simulink model "week3_problem3"  (R2020b)
settings: Solver=VariableStepAuto  StartTime=0.0  StopTime=10.0  RelTol=1e-3
model workspace (MAT data in the model file):
  Iyy = 2100
  Lf = 0.9
  Lr = 1.2
  Mb = 1200
  cf = 2500
  cr = 2000
  kf = 28000
  kr = 21000
  x0 = [-4.33578832873e-18; -0.12012244898; 6.46234853557e-27; -1.03397576569e-25]
settings Model: Creator=gokul  LastModifiedBy=gokul

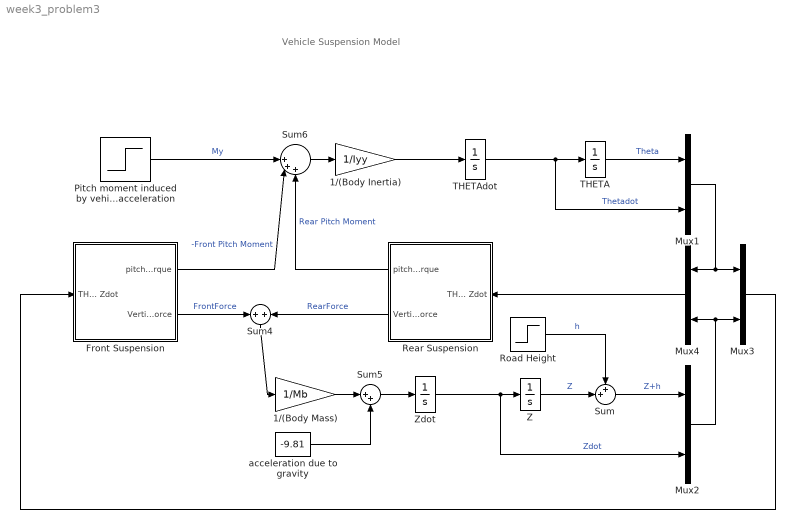
== system week3_problem3 ==
  note: Vehicle Suspension Model
  1/(Body Inertia) : Gain  Gain=1/Iyy  SaturateOnIntegerOverflow=on  OutDataTypeStr=Inherit: Same as input  ParamDataTypeStr=Inherit: Same as input
  1/(Body Mass) : Gain  Gain=1/Mb  SaturateOnIntegerOverflow=on  OutDataTypeStr=Inherit: Same as input  ParamDataTypeStr=Inherit: Same as input
  Front Suspension : Subsystem  mask(half-car suspension){K=kf, C=cf, L=-Lf}
      mask prompts: K "Stiffness = spring rate:"; C "Damping rate:"; L "Moment arm:"
      mask help:
      | Half-Car Suspension
      | The spring and damping rates for an individual wheel are entered below.  Their combined effect as applied to two wheels at the specified distance from the center of mass is computed.  The distance should be specified as positive if the subsystem is oriented such that increasing z corresponds to increasing theta, negative otherwise.
      mask Help: See "Using Simulink and Stateflow in Automotive Applications" for a mathematical derivation of the subsystem operation.  Contact your MathWorks distributor to obtain a copy.
      mask Display: plot(-1, 0, 13, 12, [1 12], [11 11], [1 5], [2 2], [1 2], [4.5 5], [2 0], [5 6], [0 2], [6 7], [2 0], [7 8], [0 1], [8 8.5], [1 1], [8.5 11], [1 1], [2 4.5], [5 5], [2 5], [4 6], [5 5], [4 4], [5 8], [6 6], [5 8], [4 6], [6.5 6.5], [5 5], [6.5 11], [0 1], [1 2], [2 3], [1 2], [4 5], [1 2])
  Mux{1..4} (4 alike) : Mux  Inputs=2
      settings: DisplayOption=signals
  Pitch moment induced by vehicle acceleration : Step  Time=3  After=100  SampleTime=0
  Rear Suspension : Subsystem  mask(half-car suspension){K=kr, C=cr, L=Lr}
      mask prompts: K "Stiffness = spring rate:"; C "Damping rate:"; L "Moment arm:"
      mask help:
      | Half-Car Suspension
      | The spring and damping rates for an individual wheel are entered below.  Their combined effect as applied to two wheels at the specified distance from the center of mass is computed.  The distance should be specified as positive if the subsystem is oriented such that increasing z corresponds to increasing theta, negative otherwise.
      mask Help: See "Using Simulink and Stateflow in Automotive Applications" for a mathematical derivation of the subsystem operation.  Contact your MathWorks distributor to obtain a copy.
      mask Display: plot(-1, 0, 13, 12, [1 12], [11 11], [1 5], [2 2], [1 2], [4.5 5], [2 0], [5 6], [0 2], [6 7], [2 0], [7 8], [0 1], [8 8.5], [1 1], [8.5 11], [1 1], [2 4.5], [5 5], [2 5], [4 6], [5 5], [4 4], [5 8], [6 6], [5 8], [4 6], [6.5 6.5], [5 5], [6.5 11], [0 1], [1 2], [2 3], [1 2], [4 5], [1 2])
  Road Height : Step  Time=7  After=0.01  SampleTime=0
  Sum : Sum  Inputs=++|
  Sum4 : Sum  InputSameDT=on  SaturateOnIntegerOverflow=on  OutDataTypeStr=Inherit: Same as first input
  Sum5 : Sum  Inputs=|++  InputSameDT=on  SaturateOnIntegerOverflow=on  OutDataTypeStr=Inherit: Same as first input
  Sum6 : Sum  Inputs=||+++  InputSameDT=on  SaturateOnIntegerOverflow=on  OutDataTypeStr=Inherit: Same as first input
  THETA : Integrator  InitialCondition=-8.7e-20
  THETAdot : Integrator  InitialCondition=8.04e-28
  Z : Integrator  InitialCondition=-0.12
  Zdot : Integrator
  acceleration due to gravity : Constant  Value=-9.81
  wires:
  Pitch moment induced by vehicle acceleration/1 -> Sum6/1  "My"
  Mux1/1 -> Mux3/1, Mux4/1
  Mux3/1 -> Front Suspension/1(THETA THETAdot Z Zdot)
  Road Height/1 -> Sum/1  "h"
  THETAdot/1 -> THETA/1, Mux1/2  "Thetadot"
  Z/1 -> Sum/2  "Z"
  Sum/1 -> Mux2/1  "Z+h"
  1/(Body Inertia)/1 -> THETAdot/1
  Mux2/1 -> Mux4/2, Mux3/2
  Sum5/1 -> Zdot/1
  Front Suspension/1(pitch Torque) -> Sum6/2  "-Front Pitch Moment"
  Mux4/1 -> Rear Suspension/1(THETA THETAdot Z Zdot)
  acceleration due to gravity/1 -> Sum5/2
  Rear Suspension/1(pitch Torque) -> Sum6/3  "Rear Pitch Moment"
  THETA/1 -> Mux1/1  "Theta"
  Front Suspension/2(Vertical Force) -> Sum4/1  "FrontForce"
  Sum6/1 -> 1/(Body Inertia)/1
  Zdot/1 -> Z/1, Mux2/2  "Zdot"
  1/(Body Mass)/1 -> Sum5/1
  Sum4/1 -> 1/(Body Mass)/1
  Rear Suspension/2(Vertical Force) -> Sum4/2  "RearForce"

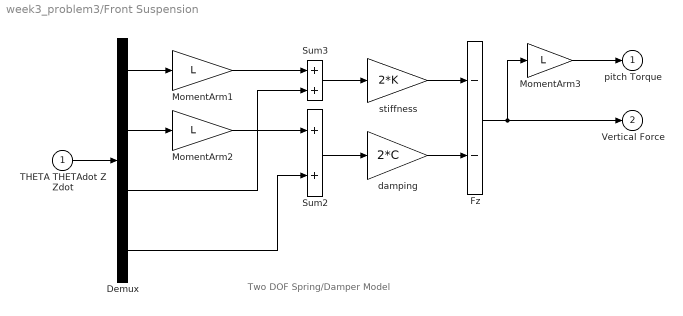
== system week3_problem3/Front Suspension ==
  note: Two DOF Spring/Damper Model
  THETA THETAdot Z Zdot : Inport
  Demux : Demux
      settings: DisplayOption=none
  Fz : Sum  Inputs=--  InputSameDT=on  SaturateOnIntegerOverflow=on  OutDataTypeStr=Inherit: Same as first input
  MomentArm1 : Gain  Gain=L  SaturateOnIntegerOverflow=on  OutDataTypeStr=Inherit: Same as input  ParamDataTypeStr=Inherit: Same as input
  MomentArm2 : Gain  Gain=L  SaturateOnIntegerOverflow=on  OutDataTypeStr=Inherit: Same as input  ParamDataTypeStr=Inherit: Same as input
  MomentArm3 : Gain  Gain=L  SaturateOnIntegerOverflow=on  OutDataTypeStr=Inherit: Same as input  ParamDataTypeStr=Inherit: Same as input
  Sum2 : Sum  InputSameDT=on  SaturateOnIntegerOverflow=on  OutDataTypeStr=Inherit: Same as first input
  Sum3 : Sum  InputSameDT=on  SaturateOnIntegerOverflow=on  OutDataTypeStr=Inherit: Same as first input
  damping : Gain  Gain=2*C  SaturateOnIntegerOverflow=on  OutDataTypeStr=Inherit: Same as input  ParamDataTypeStr=Inherit: Same as input
  stiffness : Gain  Gain=2*K  SaturateOnIntegerOverflow=on  OutDataTypeStr=Inherit: Same as input  ParamDataTypeStr=Inherit: Same as input
  pitch Torque : Outport  VectorParamsAs1DForOutWhenUnconnected=off
  Vertical Force : Outport  Port=2  VectorParamsAs1DForOutWhenUnconnected=off
  wires:
  Sum2/1 -> damping/1
  Sum3/1 -> stiffness/1
  THETA THETAdot Z Zdot/1 -> Demux/1
  damping/1 -> Fz/2
  stiffness/1 -> Fz/1
  Fz/1 -> Vertical Force/1, MomentArm3/1
  MomentArm3/1 -> pitch Torque/1
  Demux/1 -> MomentArm1/1
  Demux/2 -> MomentArm2/1
  Demux/3 -> Sum3/2
  MomentArm1/1 -> Sum3/1
  MomentArm2/1 -> Sum2/1
  Demux/4 -> Sum2/2

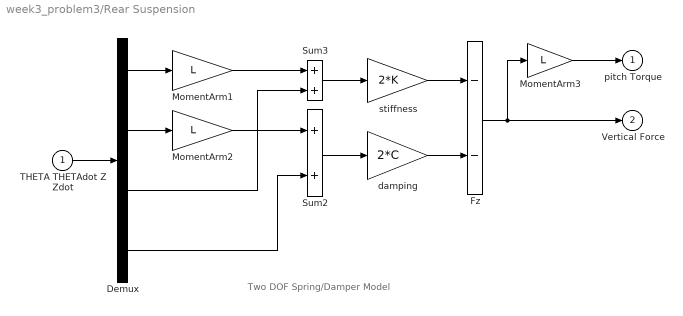
== system week3_problem3/Rear Suspension ==
  note: Two DOF Spring/Damper Model
  THETA THETAdot Z Zdot : Inport
  Demux : Demux
      settings: DisplayOption=none
  Fz : Sum  Inputs=--  InputSameDT=on  SaturateOnIntegerOverflow=on  OutDataTypeStr=Inherit: Same as first input
  MomentArm1 : Gain  Gain=L  SaturateOnIntegerOverflow=on  OutDataTypeStr=Inherit: Same as input  ParamDataTypeStr=Inherit: Same as input
  MomentArm2 : Gain  Gain=L  SaturateOnIntegerOverflow=on  OutDataTypeStr=Inherit: Same as input  ParamDataTypeStr=Inherit: Same as input
  MomentArm3 : Gain  Gain=L  SaturateOnIntegerOverflow=on  OutDataTypeStr=Inherit: Same as input  ParamDataTypeStr=Inherit: Same as input
  Sum2 : Sum  InputSameDT=on  SaturateOnIntegerOverflow=on  OutDataTypeStr=Inherit: Same as first input
  Sum3 : Sum  InputSameDT=on  SaturateOnIntegerOverflow=on  OutDataTypeStr=Inherit: Same as first input
  damping : Gain  Gain=2*C  SaturateOnIntegerOverflow=on  OutDataTypeStr=Inherit: Same as input  ParamDataTypeStr=Inherit: Same as input
  stiffness : Gain  Gain=2*K  SaturateOnIntegerOverflow=on  OutDataTypeStr=Inherit: Same as input  ParamDataTypeStr=Inherit: Same as input
  pitch Torque : Outport  VectorParamsAs1DForOutWhenUnconnected=off
  Vertical Force : Outport  Port=2  VectorParamsAs1DForOutWhenUnconnected=off
  wires:
  Demux/4 -> Sum2/2
  MomentArm2/1 -> Sum2/1
  MomentArm1/1 -> Sum3/1
  Demux/3 -> Sum3/2
  Demux/2 -> MomentArm2/1
  Demux/1 -> MomentArm1/1
  MomentArm3/1 -> pitch Torque/1
  Fz/1 -> MomentArm3/1, Vertical Force/1
  stiffness/1 -> Fz/1
  damping/1 -> Fz/2
  THETA THETAdot Z Zdot/1 -> Demux/1
  Sum3/1 -> stiffness/1
  Sum2/1 -> damping/1
